simulink model "V2X_UDP_SCLX_Control_2019b"  (R2019b)
settings: Solver=FixedStepDiscrete  StartTime=0.0  StopTime=Inf  FixedStep=0.01  RelTol=1e-3
PostLoadFcn:
  | if any(exist('dsrtsu_mdlpostloadfcn', 'file') ~= 0), dsrtsu_mdlpostloadfcn('Execute', bdroot); end
InitFcn:
  | , if any(exist('rtifpga_mdlclblib', 'file') ~= 0), rtifpga_mdlclblib('Init', bdroot); end,
  | , if any(exist('dsmpb_private', 'file') ~= 0), dsmpb_private('dsmpb_mdlclblib', 'Init', bdroot); end,
values from neighbouring files (symbols this model uses):
  CtrlZone_Length = 250    [HDVPSG_DelayComp_NewRef_RealDrop_script_case1.m]
  High_TRFC = 1    [HDVPSG_DelayComp_NewRef_RealDrop_script_case1.m]
  PSG_AMAX = 3.2    [HDVPSG_DelayComp_NewRef_RealDrop_script_case1.m]
  PSG_AMIN = -6    [HDVPSG_DelayComp_NewRef_RealDrop_script_case1.m]
  PSG_first_v0 = 13    [HDVPSG_DelayComp_NewRef_RealDrop_script_case1.m]
  PSG_HighMu_D = 15    [HDVPSG_DelayComp_NewRef_RealDrop_script_case1.m]
  PSG_HighMu_I = 125    [HDVPSG_DelayComp_NewRef_RealDrop_script_case1.m]
  PSG_HighMu_P = 75    [HDVPSG_DelayComp_NewRef_RealDrop_script_case1.m]
  PSG_HighMu_TRFC = 0.8    [HDVPSG_DelayComp_NewRef_RealDrop_script_case1.m]
  PSG_LowMu_D = 12    [HDVPSG_DelayComp_NewRef_RealDrop_script_case1.m]
  PSG_LowMu_I = 64    [HDVPSG_DelayComp_NewRef_RealDrop_script_case1.m]
  PSG_LowMu_P = 48    [HDVPSG_DelayComp_NewRef_RealDrop_script_case1.m]
  PSG_LowMu_TRFC = 0.7    [HDVPSG_DelayComp_NewRef_RealDrop_script_case1.m]
  Q_Leader = 1    [HDVPSG_DelayComp_NewRef_RealDrop_script_case1.m]
  R_Leader = 20    [HDVPSG_DelayComp_NewRef_RealDrop_script_case1.m]
  T_ADE = 0.01    [HDVPSG_DelayComp_NewRef_RealDrop_script_case1.m]
  V_MAX = 40    [HDVPSG_DelayComp_NewRef_RealDrop_script_case1.m]
  V_MIN = 0    [HDVPSG_DelayComp_NewRef_RealDrop_script_case1.m]
undefined symbols (not defined in the file or in its folder): BETA_PSG_Leader, DiscIntNeverNeededParam, UT
libraries: simulink x4, dsmpblib x3
(part 2 of 3)

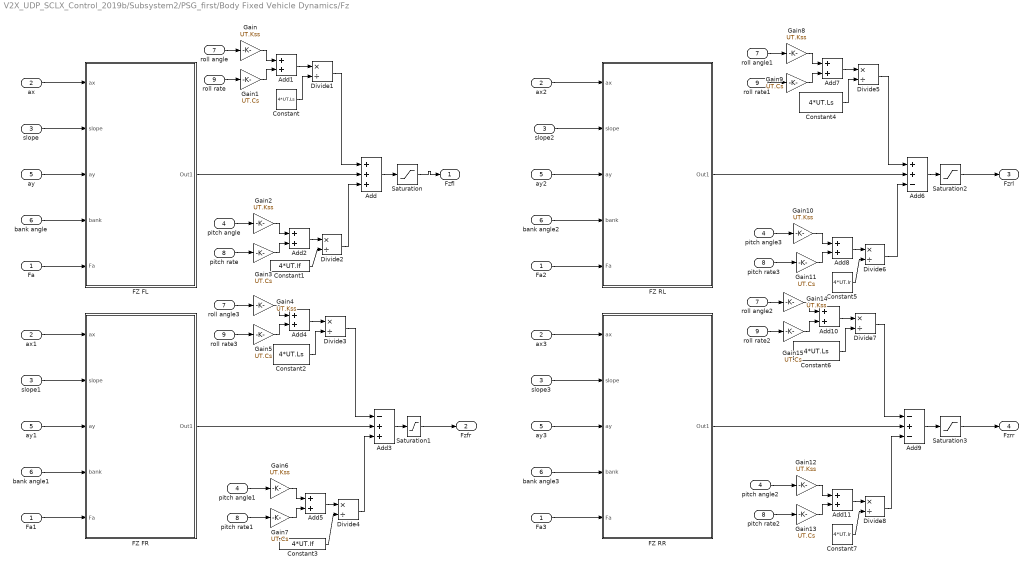
== system V2X_UDP_SCLX_Control_2019b/Subsystem2/PSG_first/Body Fixed Vehicle Dynamics/Fz ==
  Fa : Inport
  ax : Inport  Port=2
  slope : Inport  Port=3
  pitch angle : Inport  Port=4
  ay : Inport  Port=5
  bank angle : Inport  Port=6
  roll angle : Inport  Port=7
  pitch rate : Inport  Port=8
  roll rate : Inport  Port=9
  Add : Sum  Inputs=+++
  Add{1..2,4..5,7..8,10..11} (8 alike) : Sum
  Add3 : Sum  Inputs=-++
  Add6 : Sum  Inputs=++-
  Add9 : Sum  Inputs=-+-
  Constant{,2,4,6} (4 alike) : Constant  Value=4*UT.Ls
  Constant1 : Constant  Value=4*UT.lf
  Constant3 : Constant  Value=4*UT.lf
  Constant5 : Constant  Value=4*UT.lr
  Constant7 : Constant  Value=4*UT.lr
  Divide{1..8} (8 alike) : Product  Inputs=*/
  FZ FL : Subsystem
  FZ FR : Subsystem
  FZ RL : Subsystem
  FZ RR : Subsystem
  Fa1 : InportShadow
  Fa2 : InportShadow
  Fa3 : InportShadow
  Gain{,2,4,6,8,10,12,14} (8 alike) : Gain  Gain=UT.Kss
  Gain{1,3,5,7,9,11,13,15} (8 alike) : Gain  Gain=UT.Cs
  Saturation{,1..3} (4 alike) : Saturate  UpperLimit=10000  LowerLimit=100
  ax1 : InportShadow  Port=2
  ax2 : InportShadow  Port=2
  ax3 : InportShadow  Port=2
  ay1 : InportShadow  Port=5
  ay2 : InportShadow  Port=5
  ay3 : InportShadow  Port=5
  bank angle1 : InportShadow  Port=6
  bank angle2 : InportShadow  Port=6
  bank angle3 : InportShadow  Port=6
  pitch angle1 : InportShadow  Port=4
  pitch angle2 : InportShadow  Port=4
  pitch angle3 : InportShadow  Port=4
  pitch rate1 : InportShadow  Port=8
  pitch rate2 : InportShadow  Port=8
  pitch rate3 : InportShadow  Port=8
  roll angle1 : InportShadow  Port=7
  roll angle2 : InportShadow  Port=7
  roll angle3 : InportShadow  Port=7
  roll rate1 : InportShadow  Port=9
  roll rate2 : InportShadow  Port=9
  roll rate3 : InportShadow  Port=9
  slope1 : InportShadow  Port=3
  slope2 : InportShadow  Port=3
  slope3 : InportShadow  Port=3
  Fzfl : Outport  VectorParamsAs1DForOutWhenUnconnected=off
  Fzfr : Outport  Port=2  VectorParamsAs1DForOutWhenUnconnected=off
  Fzrl : Outport  Port=3  VectorParamsAs1DForOutWhenUnconnected=off
  Fzrr : Outport  Port=4  VectorParamsAs1DForOutWhenUnconnected=off
  wires:
  slope/1 -> FZ FL/2(slope)
  ax/1 -> FZ FL/1(ax)
  ay/1 -> FZ FL/3(ay)
  Fa/1 -> FZ FL/5(Fa)
  bank angle/1 -> FZ FL/4(bank)
  ay2/1 -> FZ RL/3(ay)
  slope2/1 -> FZ RL/2(slope)
  bank angle2/1 -> FZ RL/4(bank)
  ax2/1 -> FZ RL/1(ax)
  Fa2/1 -> FZ RL/5(Fa)
  slope3/1 -> FZ RR/2(slope)
  ay3/1 -> FZ RR/3(ay)
  Fa3/1 -> FZ RR/5(Fa)
  ax3/1 -> FZ RR/1(ax)
  bank angle3/1 -> FZ RR/4(bank)
  slope1/1 -> FZ FR/2(slope)
  ax1/1 -> FZ FR/1(ax)
  ay1/1 -> FZ FR/3(ay)
  bank angle1/1 -> FZ FR/4(bank)
  Fa1/1 -> FZ FR/5(Fa)
  roll angle/1 -> Gain/1
  roll rate/1 -> Gain1/1
  Gain1/1 -> Add1/2
  Gain/1 -> Add1/1
  Add1/1 -> Divide1/1
  Constant/1 -> Divide1/2
  FZ FL/1(Out1) -> Add/2
  Add/1 -> Saturation/1
  Gain3/1 -> Add2/2
  Gain2/1 -> Add2/1
  Add2/1 -> Divide2/1
  Constant1/1 -> Divide2/2
  pitch angle/1 -> Gain2/1
  pitch rate/1 -> Gain3/1
  roll angle3/1 -> Gain4/1
  roll rate3/1 -> Gain5/1
  Gain5/1 -> Add4/2
  Gain4/1 -> Add4/1
  Add4/1 -> Divide3/1
  Constant2/1 -> Divide3/2
  FZ FR/1(Out1) -> Add3/2
  Gain7/1 -> Add5/2
  Gain6/1 -> Add5/1
  Add5/1 -> Divide4/1
  Constant3/1 -> Divide4/2
  pitch angle1/1 -> Gain6/1
  pitch rate1/1 -> Gain7/1
  roll angle1/1 -> Gain8/1
  roll rate1/1 -> Gain9/1
  Gain9/1 -> Add7/2
  Gain8/1 -> Add7/1
  Add7/1 -> Divide5/1
  Constant4/1 -> Divide5/2
  FZ RL/1(Out1) -> Add6/2
  Gain11/1 -> Add8/2
  Gain10/1 -> Add8/1
  Add8/1 -> Divide6/1
  Constant5/1 -> Divide6/2
  pitch angle3/1 -> Gain10/1
  pitch rate3/1 -> Gain11/1
  roll angle2/1 -> Gain14/1
  roll rate2/1 -> Gain15/1
  Gain15/1 -> Add10/2
  Gain14/1 -> Add10/1
  Add10/1 -> Divide7/1
  Constant6/1 -> Divide7/2
  FZ RR/1(Out1) -> Add9/2
  Gain13/1 -> Add11/2
  Gain12/1 -> Add11/1
  Add11/1 -> Divide8/1
  Constant7/1 -> Divide8/2
  pitch angle2/1 -> Gain12/1
  pitch rate2/1 -> Gain13/1
  Add3/1 -> Saturation1/1
  Add6/1 -> Saturation2/1
  Add9/1 -> Saturation3/1
  Divide1/1 -> Add/1
  Divide3/1 -> Add3/1
  Divide5/1 -> Add6/1
  Divide7/1 -> Add9/1
  Saturation/1 -> Fzfl/1
  Saturation1/1 -> Fzfr/1
  Saturation2/1 -> Fzrl/1
  Saturation3/1 -> Fzrr/1
  Divide4/1 -> Add3/3
  Divide2/1 -> Add/3
  Divide8/1 -> Add9/3
  Divide6/1 -> Add6/3

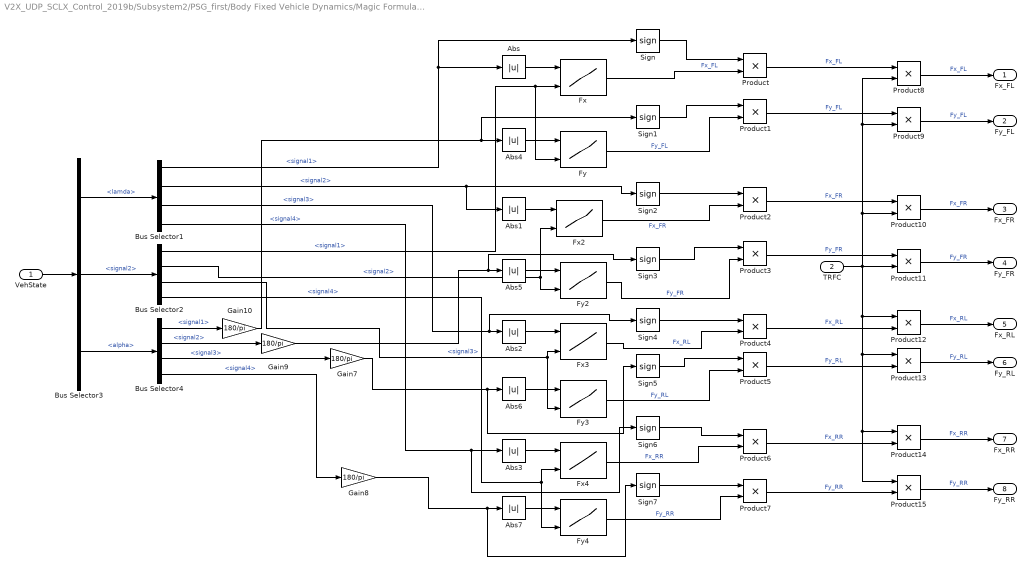
== system V2X_UDP_SCLX_Control_2019b/Subsystem2/PSG_first/Body Fixed Vehicle Dynamics/Magic Formula Tire Model1 ==
  VehState : Inport
  TRFC : Inport  Port=2
  Abs{,1..7} (8 alike) : Abs
  Bus Selector1 : BusSelector  OutputSignals=signal1,signal2,signal3,signal4
  Bus Selector2 : BusSelector  OutputSignals=signal1,signal2,signal3,signal4
  Bus Selector3 : BusSelector  OutputSignals=lamda,signal2,alpha
  Bus Selector4 : BusSelector  OutputSignals=signal1,signal2,signal3,signal4
  Fx{,2..4} (4 alike) : Lookup_n-D  BreakpointsForDimension1=[0,0.02,0.04,0.06,0.08,0.1,0.12,0.14,0.16,0.18,0.2,0.25,0.3,0.4,0.5,0.6,0.7,0.8,0.9,1]  BreakpointsForDimension2=[0,2105,3995,6120,7900,10100]  Table=reshape([0,0,0,0,0,0,0,0,0,0,0,0,0,0,0,0,0,0,0,0,0,926.741,1701.43,2240.07,2548.95,2689.78,2729.82,2717.36,2680.7,2634.75,2586.89,2476.95,2388.22,2262.94,2181.64,2125.47,2084.58,2053.55,2029.26,2029.26,0,1853.48,3402.86,4480.13,5097.92,5379.54,5459.63,5434.73,5361.4,5269.5,5173.78,4953.9,4776.46,4525.87,4363.28,4250.95,4169.16,4107.12,4058.51,4058.51,0,2780.22,5104.29,6720.21,7646.88,8069.32,8189.45,8152.09,8042.1,7904.24,7760.68,7430.85,7164.69,6788.82,6544.93,6376.42,6253.75,6160.67,6087.76,6087.76,0,3706.97,6805.72,8960.27,10195.8,10759.1,10919.3,10869.4,10722.8,10539,10347.6,9907.79,9552.92,9051.76,8726.56,8501.91,8338.33,8214.24,8117.01,8117.01,0,4633.7,8507.15,11200.3,12744.8,13448.8,13649.1,13586.8,13403.5,13173.7,12934.4,12384.7,11941.1,11314.7,10908.2,10627.4,10422.9,10267.8,10146.3,10146.3],20,6)  RndMeth=Simplest  InputSameDT=on
  Fy{,2..4} (4 alike) : Lookup_n-D  BreakpointsForDimension1=[0,0.5,1,1.5,2,2.5,3,3.5,4,4.5,5,5.5,6,6.5,7,7.5,8,8.5,9,9.5,10,12,14,16,18,20]  BreakpointsForDimension2=[0,1725,3500,6100,6950,9005]  Table=reshape([0,0,0,0,0,0,0,0,0,0,0,0,0,0,0,0,0,0,0,0,0,0,0,0,0,0,0,444.357,843.546,1162.09,1403.45,1580.72,1707.08,1795.66,1859.6,1893.83,1904.16,1896.19,1875.03,1845.3,1810.95,1775.12,1740.18,1707.8,1678.67,1653.27,1631.62,1574.53,1546.58,1531.91,1523.64,1523.64,0,894.186,1694.5,2327.41,2800.6,3142.1,3379.93,3542.12,3656.67,3713.24,3724.46,3701.92,3656.45,3597,3531.15,3464.91,3402.12,3345.23,3295.32,3252.61,3216.48,3123.37,3078,3054.18,3040.4,3040.4,0,1293.54,2452.99,3373.13,4064.18,4565.24,4915.41,5153.78,5319.43,5402.64,5422.23,5395.45,5337.38,5261.2,5177.14,5092.89,5013.56,4942.1,4879.5,4825.96,4780.78,4662.96,4604.6,4573.3,4554.99,4554.99,0,1601.93,3047.78,4214.48,5111.02,5779.43,6261.69,6599.82,6835.85,6968.31,7019.99,7011.91,6962.7,6887.9,6800.2,6709.15,6621.16,6540.06,6467.91,6405.21,6351.47,6207.67,6133.95,6093.89,6070.17,6070.17,0,1784.39,3417.9,4780.29,5873.77,6731.16,7385.32,7869.06,8215.23,8439.3,8564.79,8613.61,8605.54,8557.9,8485.17,8398.94,8308.19,8219.02,8135.36,8059.17,7991.56,7798.93,7693.72,7634.76,7599.62,7599.62],26,6)  RndMeth=Simplest  InputSameDT=on
  Gain{7..10} (4 alike) : Gain  Gain=180/pi  SaturateOnIntegerOverflow=on  SampleTime=UT.Ts_Veh  OutDataTypeStr=Inherit: Same as input  ParamDataTypeStr=Inherit: Same as input
  Product{,1..15} (16 alike) : Product
  Sign{,1..7} (8 alike) : Signum
  Fx_FL : Outport  VectorParamsAs1DForOutWhenUnconnected=off
  Fy_FL : Outport  Port=2  VectorParamsAs1DForOutWhenUnconnected=off
  Fx_FR : Outport  Port=3  VectorParamsAs1DForOutWhenUnconnected=off
  Fy_FR : Outport  Port=4  VectorParamsAs1DForOutWhenUnconnected=off
  Fx_RL : Outport  Port=5  VectorParamsAs1DForOutWhenUnconnected=off
  Fy_RL : Outport  Port=6  VectorParamsAs1DForOutWhenUnconnected=off
  Fx_RR : Outport  Port=7  VectorParamsAs1DForOutWhenUnconnected=off
  Fy_RR : Outport  Port=8  VectorParamsAs1DForOutWhenUnconnected=off
  wires:
  TRFC/1 -> Product11/2, Product10/2, Product9/2, Product8/2, Product12/1, Product13/1, Product14/1, Product15/1
  Product1/1 -> Product9/1  "Fy_FL"
  Product7/1 -> Product15/2  "Fy_RR"
  Product5/1 -> Product13/2  "Fy_RL"
  Product3/1 -> Product11/1  "Fy_FR"
  Bus Selector3/3 -> Bus Selector4/1  "<alpha>"
  Bus Selector3/2 -> Bus Selector2/1  "<signal2>"
  Bus Selector3/1 -> Bus Selector1/1  "<lamda>"
  Bus Selector4/4 -> Gain8/1  "<signal4>"
  Bus Selector4/3 -> Gain7/1  "<signal3>"
  Bus Selector4/2 -> Gain9/1  "<signal2>"
  Bus Selector4/1 -> Gain10/1  "<signal1>"
  Bus Selector1/4 -> Sign6/1, Abs3/1  "<signal4>"
  VehState/1 -> Bus Selector3/1
  Bus Selector1/1 -> Sign/1, Abs/1  "<signal1>"
  Bus Selector1/2 -> Sign2/1, Abs1/1  "<signal2>"
  Bus Selector1/3 -> Sign4/1, Abs2/1  "<signal3>"
  Abs/1 -> Fx/1
  Bus Selector2/1 -> Fy/2, Fx/2  "<signal1>"
  Abs1/1 -> Fx2/1
  Abs2/1 -> Fx3/1
  Bus Selector2/2 -> Fy2/2, Fx2/2  "<signal2>"
  Bus Selector2/3 -> Fy3/2, Fx3/2  "<signal3>"
  Abs3/1 -> Fx4/1
  Bus Selector2/4 -> Fy4/2, Fx4/2  "<signal4>"
  Abs4/1 -> Fy/1
  Abs5/1 -> Fy2/1
  Abs6/1 -> Fy3/1
  Abs7/1 -> Fy4/1
  Gain10/1 -> Sign1/1, Abs4/1
  Gain9/1 -> Sign3/1, Abs5/1
  Gain7/1 -> Sign5/1, Abs6/1
  Gain8/1 -> Sign7/1, Abs7/1
  Sign/1 -> Product/1
  Fx/1 -> Product/2  "Fx_FL"
  Product/1 -> Product8/1  "Fx_FL"
  Sign1/1 -> Product1/1
  Fy/1 -> Product1/2  "Fy_FL"
  Sign2/1 -> Product2/1
  Fx2/1 -> Product2/2  "Fx_FR"
  Product2/1 -> Product10/1  "Fx_FR"
  Sign3/1 -> Product3/1
  Fy2/1 -> Product3/2  "Fy_FR"
  Sign4/1 -> Product4/1
  Fx3/1 -> Product4/2  "Fx_RL"
  Product4/1 -> Product12/2  "Fx_RL"
  Sign5/1 -> Product5/1
  Fy3/1 -> Product5/2  "Fy_RL"
  Sign6/1 -> Product6/1
  Fx4/1 -> Product6/2  "Fx_RR"
  Product6/1 -> Product14/2  "Fx_RR"
  Sign7/1 -> Product7/1
  Fy4/1 -> Product7/2  "Fy_RR"
  Product8/1 -> Fx_FL/1  "Fx_FL"
  Product9/1 -> Fy_FL/1  "Fy_FL"
  Product10/1 -> Fx_FR/1  "Fx_FR"
  Product11/1 -> Fy_FR/1  "Fy_FR"
  Product12/1 -> Fx_RL/1  "Fx_RL"
  Product13/1 -> Fy_RL/1  "Fy_RL"
  Product14/1 -> Fx_RR/1  "Fx_RR"
  Product15/1 -> Fy_RR/1  "Fy_RR"

== system V2X_UDP_SCLX_Control_2019b/Subsystem2/PSG_first/Body Fixed Vehicle Dynamics/Tire Longitudinal Center Speed  ==
  note: Vcg
  Vx : Inport
  Vy : Inport  Port=2
  YawRate : Inport  Port=3
  VehSideSlip Beta : Inport  Port=4
  Add{,1,4,6,8} (5 alike) : Sum  SampleTime=UT.Ts_Veh
  Add2 : Sum  Inputs=+-  SampleTime=UT.Ts_Veh
  Add3 : Sum  Inputs=-+  SampleTime=UT.Ts_Veh
  Add5 : Sum  Inputs=-+  SampleTime=UT.Ts_Veh
  Add7 : Sum  Inputs=+-  SampleTime=UT.Ts_Veh
  Gain : Gain
  "Ls " : Constant  Value=UT.Ls
  Math Function : Math  Operator=square  SignedPower=on  SampleTime=UT.Ts_Veh  SaturateOnIntegerOverflow=on
  Math Function1 : Math  Operator=square  SignedPower=on  SampleTime=UT.Ts_Veh  SaturateOnIntegerOverflow=on
  Product{,1..5} (6 alike) : Product  SampleTime=UT.Ts_Veh
  Sqrt : Sqrt  SampleTime=UT.Ts_Veh  SaturateOnIntegerOverflow=on
  lf : Constant  Value=UT.lf
  lr : Constant  Value=UT.lr
  Vwfl : Outport  VectorParamsAs1DForOutWhenUnconnected=off
  Vwfr : Outport  Port=2  VectorParamsAs1DForOutWhenUnconnected=off
  Vwrl : Outport  Port=3  VectorParamsAs1DForOutWhenUnconnected=off
  Vwrr : Outport  Port=4  VectorParamsAs1DForOutWhenUnconnected=off
  wires:
  Vy/1 -> Math Function1/1
  Vx/1 -> Math Function/1
  Math Function/1 -> Add/1
  Math Function1/1 -> Add/2
  Add/1 -> Sqrt/1
  YawRate/1 -> Product5/1, Product4/1, Product2/1, Product1/1
  lf/1 -> Product/2
  VehSideSlip Beta/1 -> Gain/1
  Product/1 -> Add4/1, Add3/1
  "Ls "/1 -> Add5/2, Add6/1, Add4/2, Add3/2
  Add3/1 -> Product1/2
  Sqrt/1 -> Add8/1, Add7/1, Add1/1, Add2/1
  Product1/1 -> Add2/2
  Add2/1 -> Vwfl/1
  Add4/1 -> Product2/2
  Product2/1 -> Add1/2
  Add1/1 -> Vwfr/1
  lr/1 -> Product3/2
  Product3/1 -> Add5/1, Add6/2
  Add6/1 -> Product4/2
  Product4/1 -> Add7/2
  Add7/1 -> Vwrl/1
  Add5/1 -> Product5/2
  Product5/1 -> Add8/2
  Add8/1 -> Vwrr/1
  Gain/1 -> Product/1, Product3/1

== system V2X_UDP_SCLX_Control_2019b/Subsystem2/PSG_first/Body Fixed Vehicle Dynamics/Tire Sideslip Angle ==
  Vy : Inport
  Yaw Rate : Inport  Port=2
  Vx : Inport  Port=3
  deltaFL : Inport  Port=4
  deltaFR1 : Inport  Port=5
  Beta : Inport  Port=6
  Add : Sum  SampleTime=UT.Ts_Veh
  Add1 : Sum  Inputs=--+  SampleTime=UT.Ts_Veh
  Add2 : Sum  Inputs=-+  SampleTime=UT.Ts_Veh
  Add4 : Sum  Inputs=--+  SampleTime=UT.Ts_Veh
  Constant : Constant  Value=UT.lf
  Constant1 : Constant  Value=UT.lr
  Constant2 : Constant  Value=0.001
  Constant{3..6} (4 alike) : Constant  Value=0
  Divide : Product  Inputs=*/  SampleTime=UT.Ts_Veh
  Divide1 : Product  Inputs=/*  SampleTime=UT.Ts_Veh
  Gain{8..11} (4 alike) : Gain
  Math Function : Math  Operator=square  SignedPower=on  SampleTime=UT.Ts_Veh  SaturateOnIntegerOverflow=on
  Math Function1 : Math  Operator=square  SignedPower=on  SampleTime=UT.Ts_Veh  SaturateOnIntegerOverflow=on
  Product : Product  SampleTime=UT.Ts_Veh
  Product1 : Product  SampleTime=UT.Ts_Veh
  Saturation : Saturate  UpperLimit=1  LowerLimit=-1
  Saturation{1,3..5} (4 alike) : Saturate  UpperLimit=15*3.14/180  LowerLimit=-15*3.14/180
  Saturation2 : Saturate  UpperLimit=1  LowerLimit=-1
  Sqrt : Sqrt  SampleTime=UT.Ts_Veh  SaturateOnIntegerOverflow=on
  Switch : Switch  Criteria=u2 > Threshold
  Switch{1..4} (4 alike) : Switch  Threshold=2
  Vx{1..4} (4 alike) : InportShadow  Port=3
  Yaw Rate1 : InportShadow  Port=2
  alpha_fl: rad : Outport  VectorParamsAs1DForOutWhenUnconnected=off
  alpha_fr: rad : Outport  Port=2  VectorParamsAs1DForOutWhenUnconnected=off
  alpha_rl: rad : Outport  Port=3  VectorParamsAs1DForOutWhenUnconnected=off
  alpha_rr: rad : Outport  Port=4  VectorParamsAs1DForOutWhenUnconnected=off
  wires:
  Constant/1 -> Product/2
  Yaw Rate/1 -> Product/1
  Product/1 -> Divide/1
  Constant1/1 -> Product1/2
  Add1/1 -> Saturation/1
  Vx/1 -> Math Function1/1
  Add4/1 -> Saturation2/1
  Constant4/1 -> Switch3/3
  Vx1/1 -> Switch3/2
  Switch3/1 -> Saturation1/1
  Constant3/1 -> Switch1/3
  Vx2/1 -> Switch1/2
  Switch1/1 -> Saturation5/1
  Constant5/1 -> Switch2/3
  Vx3/1 -> Switch2/2
  Switch2/1 -> Saturation3/1
  Constant6/1 -> Switch4/3
  Vx4/1 -> Switch4/2
  Switch4/1 -> Saturation4/1
  Saturation1/1 -> Gain9/1
  Saturation5/1 -> Gain8/1
  Saturation3/1 -> Gain10/1
  Saturation4/1 -> Gain11/1
  Gain9/1 -> alpha_fl: rad/1
  Gain8/1 -> alpha_fr: rad/1
  Gain10/1 -> alpha_rl: rad/1
  Gain11/1 -> alpha_rr: rad/1
  deltaFL/1 -> Add1/3
  Math Function/1 -> Add/1
  Math Function1/1 -> Add/2
  Add/1 -> Sqrt/1
  Vy/1 -> Math Function/1
  Saturation/1 -> Switch3/1
  Divide/1 -> Add1/2, Add4/2
  deltaFR1/1 -> Add4/3
  Beta/1 -> Add2/1, Add4/1, Add1/1
  Saturation2/1 -> Switch1/1
  Divide1/1 -> Add2/2
  Add2/1 -> Switch4/1, Switch2/1
  Sqrt/1 -> Switch/2, Switch/1
  Constant2/1 -> Switch/3
  Switch/1 -> Divide/2, Divide1/1
  Product1/1 -> Divide1/2
  Yaw Rate1/1 -> Product1/1

== system V2X_UDP_SCLX_Control_2019b/Subsystem2/PSG_first/Body Fixed Vehicle Dynamics/lamda slip ratio ==
  note: used to be divided by the max of abs of wheel vel or vwcosdelta
  omegafl : Inport
  omegafr : Inport  Port=2
  omegarl : Inport  Port=3
  omegarr : Inport  Port=4
  Vwfl : Inport  Port=5
  Vwfr : Inport  Port=6
  Vwrl : Inport  Port=7
  Vwrr : Inport  Port=8
  deltaFL : Inport  Port=9
  deltaFR : Inport  Port=10
  Abs{,1..7} (8 alike) : Abs
  Constant : Constant  Value=UT.Rw
  Divide : Product  Inputs=*/  SampleTime=UT.Ts_Veh
  Divide1 : Product  Inputs=*/
  Divide2 : Product  Inputs=*/
  Divide3 : Product  Inputs=*/  SampleTime=UT.Ts_Veh
  Gain{,1..3} (4 alike) : Gain  Gain=0.1
  MinMax{,1..3} (4 alike) : MinMax  Function=max  Inputs=2
  Product{,1..5} (6 alike) : Product  SampleTime=UT.Ts_Veh
  Subtract : Sum  Inputs=+-  SampleTime=UT.Ts_Veh
  Subtract1 : Sum  Inputs=+-
  Subtract2 : Sum  Inputs=+-  SampleTime=UT.Ts_Veh
  Subtract3 : Sum  Inputs=+-  SampleTime=UT.Ts_Veh
  Trigonometric Function : Trigonometry  Operator=cos  SampleTime=UT.Ts_Veh
  Trigonometric Function1 : Trigonometry  Operator=cos
  lamdafl : Outport  VectorParamsAs1DForOutWhenUnconnected=off
  lamdafr : Outport  Port=2  VectorParamsAs1DForOutWhenUnconnected=off
  lamdarl : Outport  Port=3  VectorParamsAs1DForOutWhenUnconnected=off
  lamdarr : Outport  Port=4  VectorParamsAs1DForOutWhenUnconnected=off
  wires:
  omegafl/1 -> Product/1
  omegafr/1 -> Product1/1
  omegarl/1 -> Product2/1
  omegarr/1 -> Product3/1
  Constant/1 -> Product1/2, Product/2, Product3/2, Product2/2
  Product/1 -> Abs/1, Subtract/1
  Product1/1 -> Abs2/1, Subtract1/1
  Product2/1 -> Abs4/1, Subtract2/1
  Product3/1 -> Abs6/1, Subtract3/1
  Trigonometric Function/1 -> Product4/2
  Divide/1 -> Gain/1  "lamda_FL"
  Trigonometric Function1/1 -> Product5/2
  Vwfr/1 -> Product5/1
  Product5/1 -> Subtract1/2, Abs3/1
  Vwfl/1 -> Product4/1
  Vwrl/1 -> Abs5/1, Subtract2/2
  Subtract/1 -> Divide/1
  Subtract1/1 -> Divide1/1
  Subtract2/1 -> Divide2/1
  Subtract3/1 -> Divide3/1
  Abs/1 -> MinMax/1
  Abs1/1 -> MinMax/2
  MinMax/1 -> Divide/2
  Abs2/1 -> MinMax1/1
  Abs3/1 -> MinMax1/2
  MinMax1/1 -> Divide1/2
  Abs4/1 -> MinMax2/1
  Abs5/1 -> MinMax2/2
  MinMax2/1 -> Divide2/2
  Abs6/1 -> MinMax3/1
  Abs7/1 -> MinMax3/2
  MinMax3/1 -> Divide3/2
  Divide2/1 -> Gain2/1  "lamda_RL"
  Divide3/1 -> Gain3/1  "lamda_RR"
  Divide1/1 -> Gain1/1  "lamda_FR"
  Gain/1 -> lamdafl/1
  Gain2/1 -> lamdarl/1
  Vwrr/1 -> Abs7/1, Subtract3/2
  deltaFL/1 -> Trigonometric Function/1
  deltaFR/1 -> Trigonometric Function1/1
  Product4/1 -> Subtract/2, Abs1/1
  Gain1/1 -> lamdafr/1
  Gain3/1 -> lamdarr/1

== system V2X_UDP_SCLX_Control_2019b/Subsystem2/PSG_first/Body Fixed Vehicle Dynamics/8dof_vehicle/4tyre_torque ==
  note: -20/Rw
  Tdf : Inport
  Tbfl : Inport  Port=2
  Tbfr : Inport  Port=3
  Tbrl : Inport  Port=4
  Tbrr : Inport  Port=5
  Fxfl : Inport  Port=6
  Fxfr : Inport  Port=7
  Fxrl : Inport  Port=8
  Fxrr : Inport  Port=9
  V_ini : Inport  Port=10
  Add2 : Sum  Inputs=--+
  Add3 : Sum  Inputs=+--
  Add4 : Sum  Inputs=--
  Add5 : Sum  Inputs=--
  Constant{,1..4} (5 alike) : Constant  Value=UT.Rw
  Discrete-Time Integrator{,1..3} (4 alike) : DiscreteIntegrator  InitialConditionSource=external  InitialCondition=UT.Veh_PSG_o(7)  SampleTime=UT.Ts_Veh  ICPrevOutput=DiscIntNeverNeededParam  ICPrevScaledInput=DiscIntNeverNeededParam
  Divide{,1..3} (4 alike) : Product  Inputs=*/
  Gain{1..3,5} (4 alike) : Gain  Gain=1/UT.Jw
  Product{,1..3} (4 alike) : Product
  Saturation{,1..3} (4 alike) : Saturate  UpperLimit=100/UT.Rw  LowerLimit=-20/UT.Rw
  omega_fl : Outport  VectorParamsAs1DForOutWhenUnconnected=off
  omega_fr : Outport  Port=2  VectorParamsAs1DForOutWhenUnconnected=off
  omega_rl : Outport  Port=3  VectorParamsAs1DForOutWhenUnconnected=off
  omega_rr : Outport  Port=4  VectorParamsAs1DForOutWhenUnconnected=off
  wires:
  V_ini/1 -> Divide/1, Divide1/1, Divide2/1, Divide3/1
  Divide3/1 -> Discrete-Time Integrator3/2
  Constant4/1 -> Divide3/2
  Constant3/1 -> Divide2/2
  Divide2/1 -> Discrete-Time Integrator2/2
  Divide1/1 -> Discrete-Time Integrator1/2
  Constant2/1 -> Divide1/2
  Constant1/1 -> Divide/2
  Divide/1 -> Discrete-Time Integrator/2
  Tbrr/1 -> Add5/1
  Tbfr/1 -> Add3/2
  Product1/1 -> Add3/3
  Saturation3/1 -> omega_rr/1
  Saturation2/1 -> omega_rl/1
  Saturation1/1 -> omega_fr/1
  Saturation/1 -> omega_fl/1
  Fxrr/1 -> Product3/2
  Fxrl/1 -> Product2/2
  Fxfr/1 -> Product1/2
  Fxfl/1 -> Product/1
  Gain5/1 -> Discrete-Time Integrator/1
  Add5/1 -> Gain3/1
  Add4/1 -> Gain2/1
  Add2/1 -> Gain5/1
  Add3/1 -> Gain1/1
  Tbrl/1 -> Add4/1
  Discrete-Time Integrator3/1 -> Saturation3/1
  Discrete-Time Integrator2/1 -> Saturation2/1
  Gain2/1 -> Discrete-Time Integrator2/1
  Discrete-Time Integrator1/1 -> Saturation1/1
  Gain1/1 -> Discrete-Time Integrator1/1
  Discrete-Time Integrator/1 -> Saturation/1
  Tbfl/1 -> Add2/2
  Product2/1 -> Add4/2
  Product3/1 -> Add5/2
  Constant/1 -> Product1/1, Product2/1, Product3/1, Product/2
  Tdf/1 -> Add2/3, Add3/1
  Product/1 -> Add2/1
  Gain3/1 -> Discrete-Time Integrator3/1

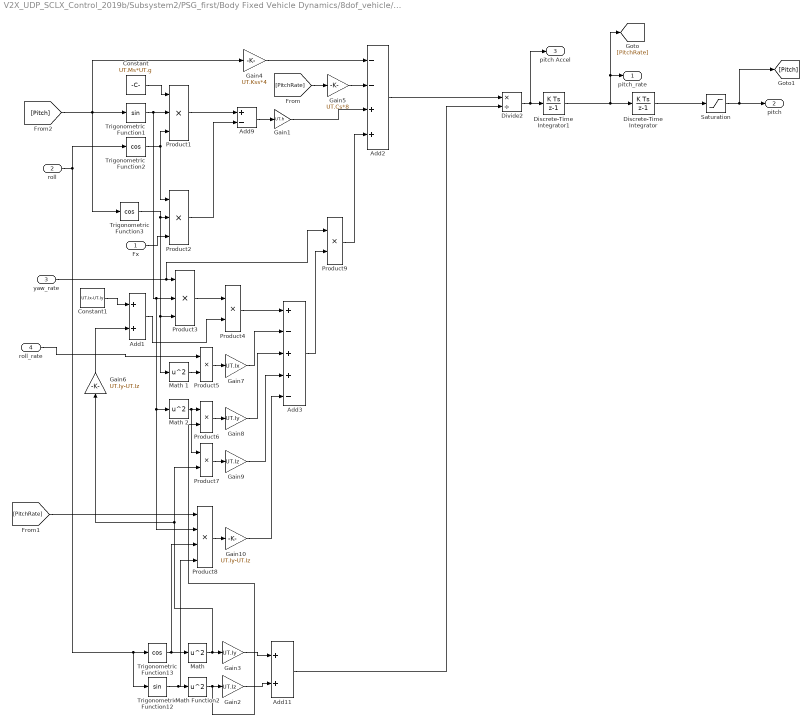
== system V2X_UDP_SCLX_Control_2019b/Subsystem2/PSG_first/Body Fixed Vehicle Dynamics/8dof_vehicle/Pitch  ==
  Fx : Inport
  roll : Inport  Port=2
  yaw_rate : Inport  Port=3
  roll_rate : Inport  Port=4
  Add1 : Sum
  Add11 : Sum
  Add2 : Sum  Inputs=--++
  Add3 : Sum  Inputs=+-++-
  Add9 : Sum  Inputs=+-
  Constant : Constant  Value=UT.Ms*UT.g
  Constant1 : Constant  Value=UT.Ix-UT.Iy
  Discrete-Time Integrator : DiscreteIntegrator  SampleTime=UT.Ts_Veh  ICPrevOutput=DiscIntNeverNeededParam  ICPrevScaledInput=DiscIntNeverNeededParam
  Discrete-Time Integrator1 : DiscreteIntegrator  SampleTime=UT.Ts_Veh  ICPrevOutput=DiscIntNeverNeededParam  ICPrevScaledInput=DiscIntNeverNeededParam
  Divide2 : Product  Inputs=*/
  Gain1 : Gain  Gain=UT.h
  Gain10 : Gain  Gain=UT.Iy-UT.Iz
  Gain2 : Gain  Gain=UT.Iz
  Gain3 : Gain  Gain=UT.Iy
  Gain4 : Gain  Gain=UT.Kss*4
  Gain5 : Gain  Gain=UT.Cs*8
  Gain6 : Gain  Gain=UT.Iy-UT.Iz
  Gain7 : Gain  Gain=UT.Ix
  Gain8 : Gain  Gain=UT.Iy
  Gain9 : Gain  Gain=UT.Iz
  "Math " : Math  Operator=square  SignedPower=on  SaturateOnIntegerOverflow=on
  Math 1 : Math  Operator=square  SignedPower=on  SaturateOnIntegerOverflow=on
  Math 2 : Math  Operator=square  SignedPower=on  SaturateOnIntegerOverflow=on
  Math Function2 : Math  Operator=square  SignedPower=on  SaturateOnIntegerOverflow=on
  Product1 : Product  Inputs=3
  Product2 : Product  Inputs=3
  Product3 : Product  Inputs=3
  Product{4..7,9} (5 alike) : Product
  Product8 : Product  Inputs=4
  Saturation : Saturate  UpperLimit=0.18  LowerLimit=-0.18
  Trigonometric Function1 : Trigonometry
  Trigonometric Function12 : Trigonometry
  Trigonometric Function13 : Trigonometry  Operator=cos
  Trigonometric Function2 : Trigonometry  Operator=cos
  Trigonometric Function3 : Trigonometry  Operator=cos
  pitch_rate : Outport  VectorParamsAs1DForOutWhenUnconnected=off
  pitch : Outport  Port=2  VectorParamsAs1DForOutWhenUnconnected=off
  pitch Accel : Outport  Port=3  VectorParamsAs1DForOutWhenUnconnected=off
  wires:
  Saturation/1 -> [Pitch], pitch/1
  Discrete-Time Integrator1/1 -> [PitchRate], pitch_rate/1, Discrete-Time Integrator/1
  roll/1 -> Trigonometric Function12/1, Trigonometric Function13/1, Trigonometric Function2/1
  Add9/1 -> Gain1/1
  Trigonometric Function13/1 -> Product8/3, "Math "/1
  "Math "/1 -> Product7/2, Gain6/1, Gain3/1
  Gain3/1 -> Add11/1
  Trigonometric Function12/1 -> Product8/4, Math Function2/1
  Gain2/1 -> Add11/2
  Add11/1 -> Divide2/2
  [Pitch] -> Gain4/1, Trigonometric Function3/1, Trigonometric Function1/1
  Constant/1 -> Product1/1
  Trigonometric Function2/1 -> Product1/3, Product2/1
  Product1/1 -> Add9/1
  Fx/1 -> Product2/3
  Trigonometric Function3/1 -> Math 1/1, Product3/3, Product2/2
  Product2/1 -> Add9/2
  Gain1/1 -> Add2/3
  Gain4/1 -> Add2/1
  Gain5/1 -> Add2/2
  Divide2/1 -> pitch Accel/1, Discrete-Time Integrator1/1
  [PitchRate] -> Gain5/1
  yaw_rate/1 -> Product9/1, Product3/1
  Product3/1 -> Product4/1
  Constant1/1 -> Add1/1
  Gain6/1 -> Add1/2
  Add1/1 -> Product4/2
  Product4/1 -> Add3/1
  roll_rate/1 -> Product5/1
  Math 1/1 -> Product5/2
  Product5/1 -> Gain7/1
  Gain7/1 -> Add3/2
  Product6/1 -> Gain8/1
  Math 2/1 -> Product7/1, Product6/1
  Trigonometric Function1/1 -> Product1/2, Product8/2, Math 2/1, Product3/2
  Gain8/1 -> Add3/3
  Math Function2/1 -> Product6/2, Gain2/1
  Product7/1 -> Gain9/1
  Gain9/1 -> Add3/4
  Product8/1 -> Gain10/1
  [PitchRate] -> Product8/1
  Gain10/1 -> Add3/5
  Add3/1 -> Product9/2
  Product9/1 -> Add2/4
  Add2/1 -> Divide2/1
  Discrete-Time Integrator/1 -> Saturation/1

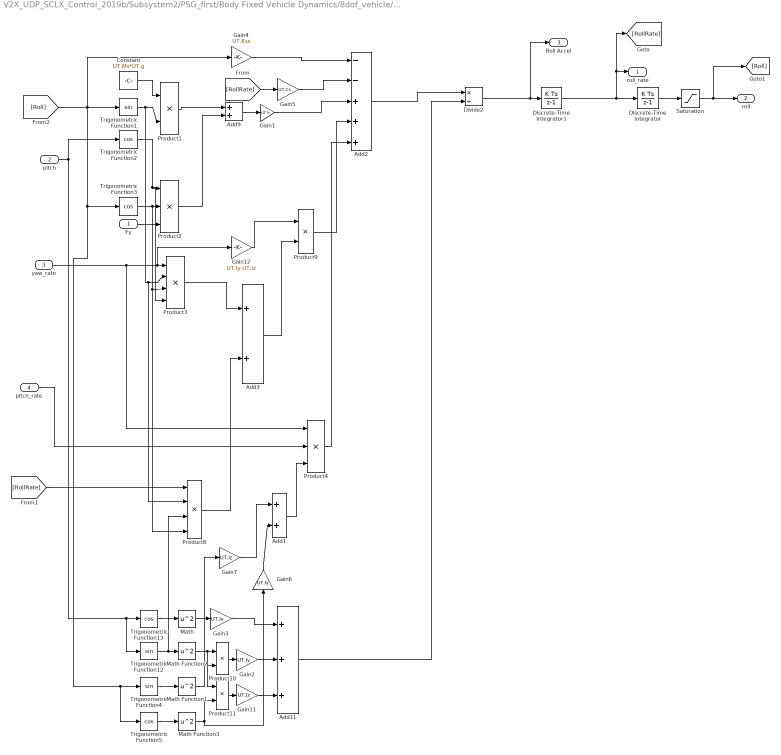
== system V2X_UDP_SCLX_Control_2019b/Subsystem2/PSG_first/Body Fixed Vehicle Dynamics/8dof_vehicle/Roll ==
  Fy : Inport
  pitch : Inport  Port=2
  yaw_rate : Inport  Port=3
  pitch_rate : Inport  Port=4
  Add1 : Sum
  Add11 : Sum  Inputs=+++
  Add2 : Sum  Inputs=--+++
  Add3 : Sum
  Add9 : Sum
  Constant : Constant  Value=UT.Ms*UT.g
  Discrete-Time Integrator : DiscreteIntegrator  SampleTime=UT.Ts_Veh  ICPrevOutput=DiscIntNeverNeededParam  ICPrevScaledInput=DiscIntNeverNeededParam
  Discrete-Time Integrator1 : DiscreteIntegrator  SampleTime=UT.Ts_Veh  ICPrevOutput=DiscIntNeverNeededParam  ICPrevScaledInput=DiscIntNeverNeededParam
  Divide2 : Product  Inputs=*/
  Gain1 : Gain  Gain=UT.h
  Gain11 : Gain  Gain=UT.Iz
  Gain12 : Gain  Gain=UT.Iy-UT.Iz
  Gain2 : Gain  Gain=UT.Iy
  Gain3 : Gain  Gain=UT.Ix
  Gain4 : Gain  Gain=UT.Kss
  Gain5 : Gain  Gain=UT.Cs
  Gain6 : Gain  Gain=UT.Iy
  Gain7 : Gain  Gain=UT.Iz
  "Math " : Math  Operator=square  SignedPower=on  SaturateOnIntegerOverflow=on
  Math Function1 : Math  Operator=square  SignedPower=on  SaturateOnIntegerOverflow=on
  Math Function2 : Math  Operator=square  SignedPower=on  SaturateOnIntegerOverflow=on
  Math Function3 : Math  Operator=square  SignedPower=on  SaturateOnIntegerOverflow=on
  Product{1,9..11} (4 alike) : Product
  Product2 : Product  Inputs=3
  Product3 : Product  Inputs=4
  Product4 : Product  Inputs=3
  Product8 : Product  Inputs=4
  Saturation : Saturate  UpperLimit=45  LowerLimit=-45
  Trigonometric Function1 : Trigonometry
  Trigonometric Function12 : Trigonometry
  Trigonometric Function{2..3,5,13} (4 alike) : Trigonometry  Operator=cos
  Trigonometric Function4 : Trigonometry
  roll_rate : Outport  VectorParamsAs1DForOutWhenUnconnected=off
  roll : Outport  Port=2  VectorParamsAs1DForOutWhenUnconnected=off
  Roll Accel : Outport  Port=3  VectorParamsAs1DForOutWhenUnconnected=off
  wires:
  Add2/1 -> Divide2/1
  Product9/1 -> Add2/4
  Add3/1 -> Product9/2
  [RollRate] -> Product8/1
  Product8/1 -> Add3/2
  Math Function2/1 -> Product11/1, Product10/1
  Trigonometric Function1/1 -> Product3/2, Product8/2, Product1/2
  Product3/1 -> Add3/1
  yaw_rate/1 -> Product4/1, Product3/1, Gain12/1
  [RollRate] -> Gain5/1
  Gain5/1 -> Add2/2
  Gain4/1 -> Add2/1
  Gain1/1 -> Add2/3
  Product2/1 -> Add9/2
  Trigonometric Function3/1 -> Product2/2, Product8/4, Product3/3
  Fy/1 -> Product2/3
  Product1/1 -> Add9/1
  Trigonometric Function2/1 -> Product3/4, Product2/1
  Constant/1 -> Product1/1
  [Roll] -> Trigonometric Function1/1, Trigonometric Function5/1, Trigonometric Function4/1, Trigonometric Function3/1, Gain4/1
  Add11/1 -> Divide2/2
  Trigonometric Function12/1 -> Product8/3, Math Function2/1
  Gain3/1 -> Add11/1
  "Math "/1 -> Gain3/1
  Trigonometric Function13/1 -> "Math "/1
  Add9/1 -> Gain1/1
  pitch/1 -> Trigonometric Function2/1, Trigonometric Function13/1, Trigonometric Function12/1
  Discrete-Time Integrator/1 -> Saturation/1
  Saturation/1 -> roll/1, [Roll]
  Product10/1 -> Gain2/1
  Trigonometric Function4/1 -> Math Function1/1
  Math Function1/1 -> Gain7/1, Product10/2
  Gain2/1 -> Add11/2
  Gain11/1 -> Add11/3
  Product11/1 -> Gain11/1
  Trigonometric Function5/1 -> Math Function3/1
  Math Function3/1 -> Product11/2, Gain6/1
  Gain12/1 -> Product9/1
  pitch_rate/1 -> Product4/2
  Gain6/1 -> Add1/2
  Gain7/1 -> Add1/1
  Add1/1 -> Product4/3
  Product4/1 -> Add2/5
  Divide2/1 -> Roll Accel/1, Discrete-Time Integrator1/1
  Discrete-Time Integrator1/1 -> Discrete-Time Integrator/1, roll_rate/1, [RollRate]

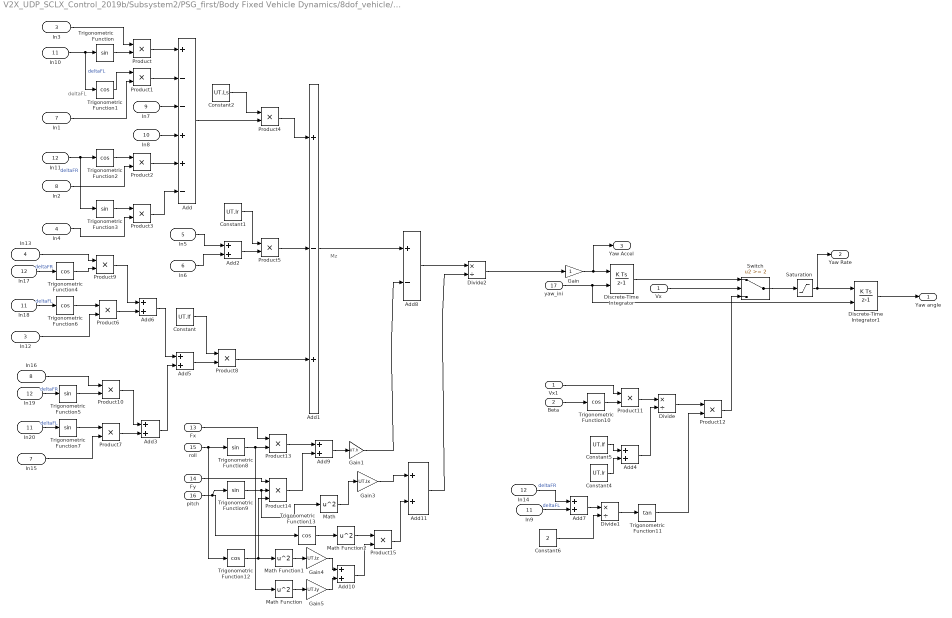
== system V2X_UDP_SCLX_Control_2019b/Subsystem2/PSG_first/Body Fixed Vehicle Dynamics/8dof_vehicle/Yaw Dynamics ==
  note: Mz
  note: deltaFL
  Vx : Inport
  Beta : Inport  Port=2
  In3 : Inport  Port=3
  In4 : Inport  Port=4
  In5 : Inport  Port=5
  In6 : Inport  Port=6
  In1 : Inport  Port=7
  In2 : Inport  Port=8
  In7 : Inport  Port=9
  In8 : Inport  Port=10
  In10 : Inport  Port=11
  In11 : Inport  Port=12
  Fx : Inport  Port=13
  Fy : Inport  Port=14
  roll : Inport  Port=15
  "pitch " : Inport  Port=16
  yaw_ini : Inport  Port=17
  Add : Sum  Inputs=+--++-
  Add1 : Sum  Inputs=+-+
  Add{2..7,9..11} (9 alike) : Sum
  Add8 : Sum  Inputs=+-
  Constant : Constant  Value=UT.lf
  Constant1 : Constant  Value=UT.lr
  Constant2 : Constant  Value=UT.Ls
  Constant4 : Constant  Value=UT.lr
  Constant5 : Constant  Value=UT.lf
  Constant6 : Constant  Value=2
  Discrete-Time Integrator : DiscreteIntegrator  InitialConditionSource=external  InitialCondition=UT.Veh_PSG_o(3)  SampleTime=UT.Ts_Veh  ICPrevOutput=DiscIntNeverNeededParam  ICPrevScaledInput=DiscIntNeverNeededParam
  Discrete-Time Integrator1 : DiscreteIntegrator  InitialConditionSource=external  InitialCondition=UT.Veh_PSG_o(3)  SampleTime=UT.Ts_Veh  ICPrevOutput=DiscIntNeverNeededParam  ICPrevScaledInput=DiscIntNeverNeededParam
  Divide : Product  Inputs=*/
  Divide1 : Product  Inputs=*/
  Divide2 : Product  Inputs=*/
  Gain : Gain
  Gain1 : Gain  Gain=UT.h
  Gain3 : Gain  Gain=UT.Ix
  Gain4 : Gain  Gain=UT.Iz
  Gain5 : Gain  Gain=UT.Iy
  In12 : InportShadow  Port=3
  In13 : InportShadow  Port=4
  In14 : InportShadow  Port=12
  In15 : InportShadow  Port=7
  In16 : InportShadow  Port=8
  In17 : InportShadow  Port=12
  In18 : InportShadow  Port=11
  In19 : InportShadow  Port=12
  In20 : InportShadow  Port=11
  In9 : InportShadow  Port=11
  "Math " : Math  Operator=square  SignedPower=on  SaturateOnIntegerOverflow=on
  Math Function : Math  Operator=square  SignedPower=on  SaturateOnIntegerOverflow=on
  Math Function1 : Math  Operator=square  SignedPower=on  SaturateOnIntegerOverflow=on
  Math Function2 : Math  Operator=square  SignedPower=on  SaturateOnIntegerOverflow=on
  Product{,1..13,15} (15 alike) : Product
  Product14 : Product  Inputs=3
  Saturation : Saturate  UpperLimit=50*3.14/180  LowerLimit=-50*3.14/180  SampleTime=UT.Ts_Veh
  Switch : Switch  Threshold=2
  Trigonometric Function{,3,5,7..9} (6 alike) : Trigonometry
  Trigonometric Function{1..2,4,6,10,12..13} (7 alike) : Trigonometry  Operator=cos
  Trigonometric Function11 : Trigonometry  Operator=tan
  Vx1 : InportShadow
  Yaw angle : Outport  VectorParamsAs1DForOutWhenUnconnected=off
  Yaw Rate : Outport  Port=2  VectorParamsAs1DForOutWhenUnconnected=off
  Yaw Accel : Outport  Port=3  VectorParamsAs1DForOutWhenUnconnected=off
  wires:
  yaw_ini/1 -> Discrete-Time Integrator1/2, Discrete-Time Integrator/2
  Discrete-Time Integrator/1 -> Switch/1
  Discrete-Time Integrator1/1 -> Yaw angle/1
  Gain/1 -> Yaw Accel/1, Discrete-Time Integrator/1
  Vx/1 -> Switch/2
  Constant4/1 -> Add4/2
  Constant5/1 -> Add4/1
  Add4/1 -> Divide/2
  Add7/1 -> Divide1/1
  Constant6/1 -> Divide1/2
  Beta/1 -> Trigonometric Function10/1
  Vx1/1 -> Product11/1
  Trigonometric Function10/1 -> Product11/2
  Product11/1 -> Divide/1
  Divide1/1 -> Trigonometric Function11/1
  Trigonometric Function11/1 -> Product12/2
  Divide/1 -> Product12/1
  Switch/1 -> Saturation/1
  Product12/1 -> Switch/3
  Saturation/1 -> Discrete-Time Integrator1/1, Yaw Rate/1
  In10/1 -> Trigonometric Function1/1, Trigonometric Function/1  "deltaFL"
  In3/1 -> Product/1
  Trigonometric Function/1 -> Product/2
  Product/1 -> Add/1
  Trigonometric Function1/1 -> Product1/1
  In1/1 -> Product1/2
  Product1/1 -> Add/2
  In7/1 -> Add/3
  In8/1 -> Add/4
  Trigonometric Function2/1 -> Product2/1
  In2/1 -> Product2/2
  Product2/1 -> Add/5
  Trigonometric Function3/1 -> Product3/1
  In4/1 -> Product3/2
  Product3/1 -> Add/6
  Add/1 -> Product4/2
  Constant2/1 -> Product4/1
  Product4/1 -> Add1/1
  In5/1 -> Add2/1
  In6/1 -> Add2/2
  Add2/1 -> Product5/2
  Constant1/1 -> Product5/1
  Product5/1 -> Add1/2
  In13/1 -> Product9/1
  Add1/1 -> Add8/1
  Add6/1 -> Add5/1
  Add5/1 -> Product8/2
  Constant/1 -> Product8/1
  Product8/1 -> Add1/3
  In11/1 -> Trigonometric Function3/1, Trigonometric Function2/1  "deltaFR"
  In12/1 -> Product6/2
  Product9/1 -> Add6/1
  Product6/1 -> Add6/2
  Trigonometric Function4/1 -> Product9/2
  Trigonometric Function6/1 -> Product6/1
  In18/1 -> Trigonometric Function6/1  "deltaFL"
  In17/1 -> Trigonometric Function4/1  "deltaFR"
  In16/1 -> Product10/1
  Add3/1 -> Add5/2
  In15/1 -> Product7/2
  Product10/1 -> Add3/1
  Product7/1 -> Add3/2
  Trigonometric Function5/1 -> Product10/2
  Trigonometric Function7/1 -> Product7/1
  In19/1 -> Trigonometric Function5/1  "deltaFR"
  In20/1 -> Trigonometric Function7/1  "deltaFL"
  In9/1 -> Add7/2  "deltaFL"
  In14/1 -> Add7/1  "deltaFR"
  roll/1 -> Trigonometric Function8/1, Trigonometric Function12/1
  Trigonometric Function8/1 -> Math Function/1, Product13/2
  Fx/1 -> Product13/1
  Product13/1 -> Add9/1
  Fy/1 -> Product14/1
  "pitch "/1 -> Trigonometric Function9/1, Trigonometric Function13/1
  Trigonometric Function9/1 -> "Math "/1, Product14/2
  Trigonometric Function12/1 -> Product14/3, Math Function1/1
  Product14/1 -> Add9/2
  Add9/1 -> Gain1/1
  Gain1/1 -> Add8/2
  Add8/1 -> Divide2/1
  Math Function/1 -> Gain5/1
  Gain5/1 -> Add10/2
  Math Function1/1 -> Gain4/1
  Gain4/1 -> Add10/1
  Add10/1 -> Product15/2
  Trigonometric Function13/1 -> Math Function2/1
  Math Function2/1 -> Product15/1
  Product15/1 -> Add11/2
  Gain3/1 -> Add11/1
  "Math "/1 -> Gain3/1
  Add11/1 -> Divide2/2
  Divide2/1 -> Gain/1

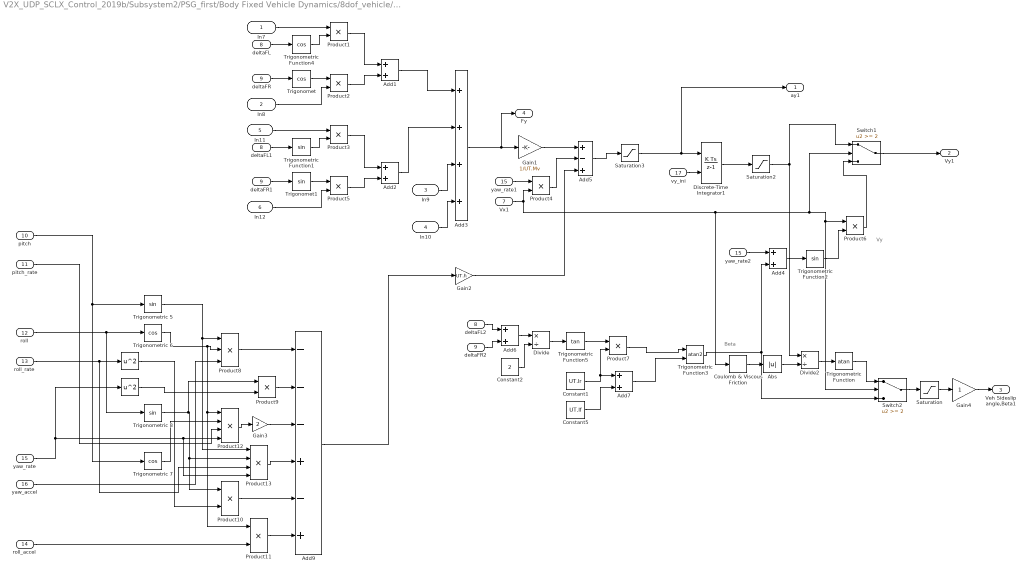
== system V2X_UDP_SCLX_Control_2019b/Subsystem2/PSG_first/Body Fixed Vehicle Dynamics/8dof_vehicle/lateral ==
  note: Beta
  note: Vy
  In7 : Inport
  In8 : Inport  Port=2
  In9 : Inport  Port=3
  In10 : Inport  Port=4
  In11 : Inport  Port=5
  In12 : Inport  Port=6
  Vx1 : Inport  Port=7
  deltaFL : Inport  Port=8
  deltaFR : Inport  Port=9
  pitch : Inport  Port=10
  pitch_rate : Inport  Port=11
  roll : Inport  Port=12
  roll_rate : Inport  Port=13
  roll_accel : Inport  Port=14
  yaw_rate : Inport  Port=15
  yaw_accel : Inport  Port=16
  vy_ini : Inport  Port=17
  " " : Math  Operator=square  SignedPower=on  SaturateOnIntegerOverflow=on
  " " : Math  Operator=square  SignedPower=on  SaturateOnIntegerOverflow=on
  Abs : Abs
  Add{1..2,4,6..7} (5 alike) : Sum
  Add3 : Sum  Inputs=++++
  Add5 : Sum  Inputs=+-+
  Add9 : Sum  Inputs=---+-+
  Constant1 : Constant  Value=UT.lr
  Constant2 : Constant  Value=2
  Constant5 : Constant  Value=UT.lf
  Coulomb & Viscous Friction : simulink/Discontinuities/Coulomb & Viscous Friction  offset=0.01  gain=1
  Discrete-Time Integrator1 : DiscreteIntegrator  InitialConditionSource=external  InitialCondition=UT.Veh_PSG_o(2)  SampleTime=UT.Ts_Veh  ICPrevOutput=DiscIntNeverNeededParam  ICPrevScaledInput=DiscIntNeverNeededParam
  Divide : Product  Inputs=*/
  Divide2 : Product  Inputs=*/
  Gain1 : Gain  Gain=1/UT.Mv
  Gain2 : Gain  Gain=UT.h
  Gain3 : Gain  Gain=2
  Gain4 : Gain
  Product{1..3,5..7,9..11} (9 alike) : Product
  Product12 : Product  Inputs=4
  Product13 : Product  Inputs=4
  Product4 : Product  RndMeth=Zero
  Product8 : Product  Inputs=3
  Saturation : Saturate  UpperLimit=10*3.14/180  LowerLimit=-10*3.14/180
  Saturation2 : Saturate  UpperLimit=100  LowerLimit=-100
  Saturation3 : Saturate  UpperLimit=6  LowerLimit=-6
  Switch1 : Switch  Threshold=2
  Switch2 : Switch  Threshold=2
  Trigonomet : Trigonometry  Operator=cos
  Trigonomet1 : Trigonometry
  Trigonometric 5 : Trigonometry
  Trigonometric 6 : Trigonometry  Operator=cos
  Trigonometric 7 : Trigonometry  Operator=cos
  Trigonometric 8 : Trigonometry
  Trigonometric Function : Trigonometry  Operator=atan
  Trigonometric Function1 : Trigonometry
  Trigonometric Function2 : Trigonometry
  Trigonometric Function3 : Trigonometry  Operator=atan2
  Trigonometric Function4 : Trigonometry  Operator=cos
  Trigonometric Function5 : Trigonometry  Operator=tan
  deltaFL1 : InportShadow  Port=8
  deltaFL2 : InportShadow  Port=8
  deltaFR1 : InportShadow  Port=9
  deltaFR2 : InportShadow  Port=9
  yaw_rate1 : InportShadow  Port=15
  yaw_rate2 : InportShadow  Port=15
  ay1 : Outport  VectorParamsAs1DForOutWhenUnconnected=off
  Vy1 : Outport  Port=2  VectorParamsAs1DForOutWhenUnconnected=off
  Veh Sideslip angle,Beta1 : Outport  Port=3  VectorParamsAs1DForOutWhenUnconnected=off
  Fy : Outport  Port=4  VectorParamsAs1DForOutWhenUnconnected=off
  wires:
  vy_ini/1 -> Discrete-Time Integrator1/2
  Gain1/1 -> Add5/1
  Add5/1 -> Saturation3/1
  In7/1 -> Product1/1
  In8/1 -> Product2/2
  yaw_rate1/1 -> Product4/1
  Add1/1 -> Add3/1
  In9/1 -> Add3/3
  In10/1 -> Add3/4
  Product4/1 -> Add5/2
  Discrete-Time Integrator1/1 -> Saturation2/1
  Trigonomet/1 -> Product2/1
  Trigonometric Function4/1 -> Product1/2
  deltaFL/1 -> Trigonometric Function4/1
  deltaFR/1 -> Trigonomet/1
  Product1/1 -> Add1/1
  Product2/1 -> Add1/2
  In11/1 -> Product3/1
  In12/1 -> Product5/2
  Trigonomet1/1 -> Product5/1
  Trigonometric Function1/1 -> Product3/2
  Product3/1 -> Add2/1
  Product5/1 -> Add2/2
  Add2/1 -> Add3/2
  deltaFL1/1 -> Trigonometric Function1/1
  deltaFR1/1 -> Trigonomet1/1
  yaw_rate2/1 -> Add4/1
  Add4/1 -> Trigonometric Function2/1
  Trigonometric Function2/1 -> Product6/2
  deltaFL2/1 -> Add6/1
  deltaFR2/1 -> Add6/2
  Add6/1 -> Divide/1
  Constant2/1 -> Divide/2
  Divide/1 -> Trigonometric Function5/1
  Trigonometric Function5/1 -> Product7/1
  Constant1/1 -> Product7/2, Add7/1
  Product7/1 -> Trigonometric Function3/1
  Constant5/1 -> Add7/2
  Saturation2/1 -> Divide2/1, Switch1/1
  Product6/1 -> Switch1/3
  Divide2/1 -> Trigonometric Function/1
  Trigonometric Function3/1 -> Add4/2, Switch2/3
  Vx1/1 -> Product4/2, Coulomb & Viscous Friction/1, Product6/1, Switch2/2, Switch1/2
  Abs/1 -> Divide2/2
  Add7/1 -> Trigonometric Function3/2
  Switch2/1 -> Saturation/1
  Saturation/1 -> Gain4/1
  Gain2/1 -> Add5/3
  pitch_rate/1 -> Product12/3
  roll_rate/1 -> Product13/3, " "/1
  yaw_rate/1 -> Product13/4, Product12/4, " "/1
  yaw_accel/1 -> Product8/3
  pitch/1 -> Trigonometric 7/1, Trigonometric 5/1
  roll/1 -> Trigonometric 8/1, Trigonometric 6/1
  Trigonometric 6/1 -> Product11/1, Product12/1, Product8/2
  Trigonometric 5/1 -> Product13/1, Product8/1
  Product8/1 -> Add9/1
  Product9/1 -> Add9/2
  Product12/1 -> Gain3/1
  Gain3/1 -> Add9/3
  Trigonometric 7/1 -> Product12/2
  Product13/1 -> Add9/4
  Product10/1 -> Add9/5
  Trigonometric 8/1 -> Product9/1, Product13/2, Product10/1
  Product11/1 -> Add9/6
  " "/1 -> Product9/2
  " "/1 -> Product10/2
  roll_accel/1 -> Product11/2
  Trigonometric Function/1 -> Switch2/1
  Add3/1 -> Fy/1, Gain1/1
  Add9/1 -> Gain2/1
  Gain4/1 -> Veh Sideslip angle,Beta1/1
  Saturation3/1 -> Discrete-Time Integrator1/1, ay1/1
  Switch1/1 -> Vy1/1
  Coulomb & Viscous Friction/1 -> Abs/1

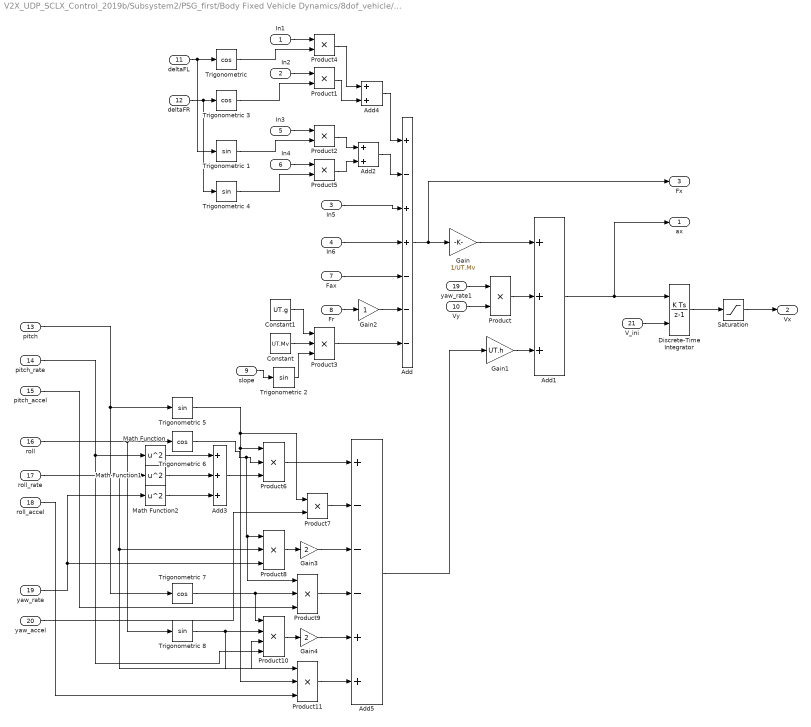
== system V2X_UDP_SCLX_Control_2019b/Subsystem2/PSG_first/Body Fixed Vehicle Dynamics/8dof_vehicle/longitudinal ==
  In1 : Inport
  In2 : Inport  Port=2
  In5 : Inport  Port=3
  In6 : Inport  Port=4
  In3 : Inport  Port=5
  In4 : Inport  Port=6
  Fax : Inport  Port=7
  Fr : Inport  Port=8
  slope : Inport  Port=9
  Vy : Inport  Port=10
  deltaFL : Inport  Port=11
  deltaFR : Inport  Port=12
  pitch : Inport  Port=13
  pitch_rate : Inport  Port=14
  pitch_accel : Inport  Port=15
  roll : Inport  Port=16
  roll_rate : Inport  Port=17
  roll_accel : Inport  Port=18
  yaw_rate : Inport  Port=19
  yaw_accel : Inport  Port=20
  V_ini : Inport  Port=21
  Add : Sum  Inputs=+-++---
  Add1 : Sum  Inputs=+++
  Add2 : Sum
  Add3 : Sum  Inputs=+++
  Add4 : Sum
  Add5 : Sum  Inputs=+---++
  Constant : Constant  Value=UT.Mv
  Constant1 : Constant  Value=UT.g
  Discrete-Time Integrator : DiscreteIntegrator  InitialConditionSource=external  InitialCondition=UT.Veh_PSG_o(1)  SampleTime=UT.Ts_Veh  ICPrevOutput=DiscIntNeverNeededParam  ICPrevScaledInput=DiscIntNeverNeededParam
  Gain : Gain  Gain=1/UT.Mv
  Gain1 : Gain  Gain=UT.h
  Gain2 : Gain
  Gain3 : Gain  Gain=2
  Gain4 : Gain  Gain=2
  Math Function : Math  Operator=square  SignedPower=on  SaturateOnIntegerOverflow=on
  Math Function1 : Math  Operator=square  SignedPower=on  SaturateOnIntegerOverflow=on
  Math Function2 : Math  Operator=square  SignedPower=on  SaturateOnIntegerOverflow=on
  Product{,1..2,4..5,7} (6 alike) : Product
  Product10 : Product  Inputs=4
  Product{3,6,8..9,11} (5 alike) : Product  Inputs=3
  Saturation : Saturate  UpperLimit=50  LowerLimit=0
  Trigonometric {,3,6..7} (4 alike) : Trigonometry  Operator=cos
  Trigonometric {1..2,4..5,8} (5 alike) : Trigonometry
  yaw_rate1 : InportShadow  Port=19
  ax : Outport  VectorParamsAs1DForOutWhenUnconnected=off
  Vx : Outport  Port=2  VectorParamsAs1DForOutWhenUnconnected=off
  Fx : Outport  Port=3  VectorParamsAs1DForOutWhenUnconnected=off
  wires:
  V_ini/1 -> Discrete-Time Integrator/2
  Discrete-Time Integrator/1 -> Saturation/1
  Fax/1 -> Add/5
  Fr/1 -> Gain2/1
  slope/1 -> Trigonometric 2/1
  Product3/1 -> Add/7
  yaw_rate1/1 -> Product/1
  Vy/1 -> Product/2
  Add/1 -> Fx/1, Gain/1
  Product/1 -> Add1/2
  Gain/1 -> Add1/1
  In1/1 -> Product4/1
  Product4/1 -> Add4/1
  Add4/1 -> Add/1
  In3/1 -> Product2/1
  In4/1 -> Product5/1
  Add2/1 -> Add/2
  In5/1 -> Add/3
  In6/1 -> Add/4
  Add1/1 -> Discrete-Time Integrator/1, ax/1
  Trigonometric 2/1 -> Product3/3
  Constant1/1 -> Product3/1
  Constant/1 -> Product3/2
  Gain2/1 -> Add/6
  Product1/1 -> Add4/2
  In2/1 -> Product1/1
  deltaFL/1 -> Trigonometric 1/1, "Trigonometric "/1
  "Trigonometric "/1 -> Product4/2
  deltaFR/1 -> Trigonometric 4/1, Trigonometric 3/1
  Trigonometric 3/1 -> Product1/2
  Trigonometric 1/1 -> Product2/2
  Trigonometric 4/1 -> Product5/2
  Product2/1 -> Add2/1
  Product5/1 -> Add2/2
  Saturation/1 -> Vx/1
  Gain1/1 -> Add1/3
  pitch_rate/1 -> Product10/4, Math Function/1
  roll_rate/1 -> Product10/3, Product8/2, Math Function1/1
  yaw_rate/1 -> Product8/3, Math Function2/1
  Math Function/1 -> Add3/1
  Math Function1/1 -> Add3/2
  Math Function2/1 -> Add3/3
  Add3/1 -> Product6/3
  pitch/1 -> Trigonometric 7/1, Trigonometric 5/1
  roll/1 -> Trigonometric 8/1, Trigonometric 6/1
  Trigonometric 6/1 -> Product9/1, Product8/1, Product6/2
  Trigonometric 5/1 -> Product7/1, Product11/2, Product6/1
  Product6/1 -> Add5/1
  yaw_accel/1 -> Product7/2
  Product7/1 -> Add5/2
  Product8/1 -> Gain3/1
  Gain3/1 -> Add5/3
  Trigonometric 7/1 -> Product10/1, Product9/2
  pitch_accel/1 -> Product9/3
  Product9/1 -> Add5/4
  Gain4/1 -> Add5/5
  Product10/1 -> Gain4/1
  Trigonometric 8/1 -> Product11/1, Product10/2
  Product11/1 -> Add5/6
  roll_accel/1 -> Product11/3
  Add5/1 -> Gain1/1

== system V2X_UDP_SCLX_Control_2019b/Subsystem2/PSG_first/Body Fixed Vehicle Dynamics/Driving Resistance Subsystem/Aerodynamic Resistance ==
  note: Fa=0.5*p*Cd*A(Vx+Vw)^2
  note: Vx=m/s
  note: increaesd to 0.75*...
  Vx : Inport
  X Aerodynamic Fcn : Fcn  Expr=0.75*UT.rho*UT.Cd*UT.Awind*(u(1)+UT.Vw)^2  SampleTime=UT.Ts_Veh
  Fa : Outport  VectorParamsAs1DForOutWhenUnconnected=off
  wires:
  X Aerodynamic Fcn/1 -> Fa/1
  Vx/1 -> X Aerodynamic Fcn/1

== system V2X_UDP_SCLX_Control_2019b/Subsystem2/PSG_first/Body Fixed Vehicle Dynamics/Driving Resistance Subsystem/Rolling resistance ==
  note: added *2
  Vx : Inport
  Rolling resistance Fcn1 : Fcn  Expr=(0.005+(1/2.013)*(0.01+0.0095*((3.6*u(1))/100)^2))*UT.Mv*UT.g*2  SampleTime=UT.Ts_Veh
  Fr : Outport  VectorParamsAs1DForOutWhenUnconnected=off
  wires:
  Vx/1 -> Rolling resistance Fcn1/1
  Rolling resistance Fcn1/1 -> Fr/1

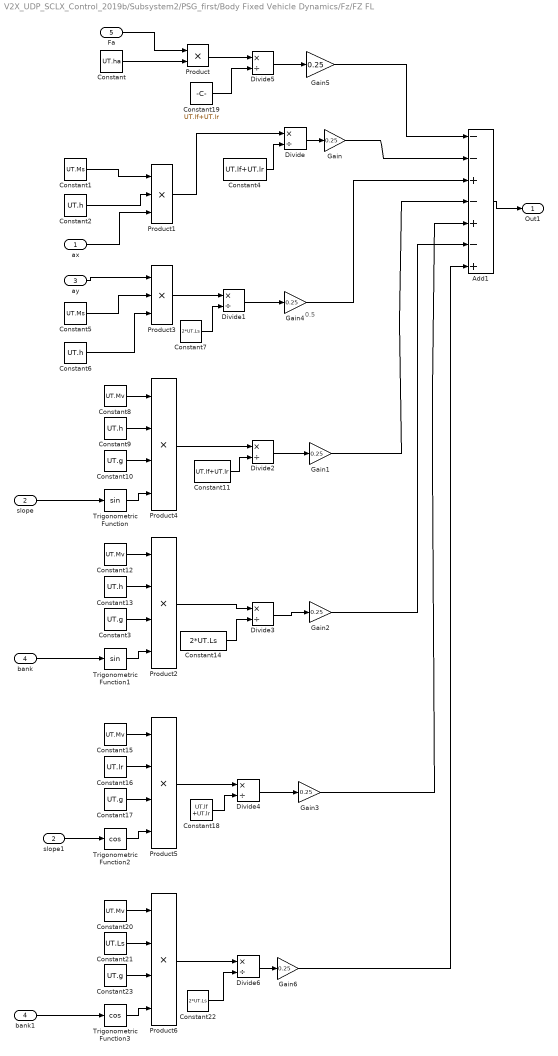
== system V2X_UDP_SCLX_Control_2019b/Subsystem2/PSG_first/Body Fixed Vehicle Dynamics/Fz/FZ FL ==
  note: 0.5
  ax : Inport
  slope : Inport  Port=2
  ay : Inport  Port=3
  bank : Inport  Port=4
  Fa : Inport  Port=5
  Add1 : Sum  Inputs=--+-+-+
  Constant : Constant  Value=UT.ha
  Constant1 : Constant  Value=UT.Ms
  Constant{3,10,17,23} (4 alike) : Constant  Value=UT.g
  Constant11 : Constant  Value=UT.lf+UT.lr
  Constant{8,12,15,20} (4 alike) : Constant  Value=UT.Mv
  Constant{2,6,9,13} (4 alike) : Constant  Value=UT.h
  Constant14 : Constant  Value=2*UT.Ls
  Constant16 : Constant  Value=UT.lr
  Constant18 : Constant  Value=UT.lf +UT.lr
  Constant19 : Constant  Value=UT.lf+UT.lr
  Constant21 : Constant  Value=UT.Ls
  Constant22 : Constant  Value=2*UT.Ls
  Constant4 : Constant  Value=UT.lf+UT.lr
  Constant5 : Constant  Value=UT.Ms
  Constant7 : Constant  Value=2*UT.Ls
  Divide{,1..6} (7 alike) : Product  Inputs=*/
  Gain{,1..6} (7 alike) : Gain  Gain=0.25
  Product : Product
  Product1 : Product  Inputs=3
  Product{2,4..6} (4 alike) : Product  Inputs=4
  Product3 : Product  Inputs=3
  Trigonometric Function : Trigonometry
  Trigonometric Function1 : Trigonometry
  Trigonometric Function2 : Trigonometry  Operator=cos
  Trigonometric Function3 : Trigonometry  Operator=cos
  bank1 : InportShadow  Port=4
  slope1 : InportShadow  Port=2
  Out1 : Outport  VectorParamsAs1DForOutWhenUnconnected=off
  wires:
  Constant1/1 -> Product1/1
  Constant2/1 -> Product1/2
  ax/1 -> Product1/3
  Constant4/1 -> Divide/2
  ay/1 -> Product3/1
  Constant5/1 -> Product3/2
  Constant6/1 -> Product3/3
  Product3/1 -> Divide1/1
  Constant7/1 -> Divide1/2
  Divide/1 -> Gain/1
  Divide1/1 -> Gain4/1
  Constant8/1 -> Product4/1
  Constant9/1 -> Product4/2
  Constant10/1 -> Product4/3
  slope/1 -> Trigonometric Function/1
  Trigonometric Function/1 -> Product4/4
  Constant11/1 -> Divide2/2
  Divide2/1 -> Gain1/1
  Product4/1 -> Divide2/1
  Constant12/1 -> Product2/1
  Constant13/1 -> Product2/2
  Constant3/1 -> Product2/3
  bank/1 -> Trigonometric Function1/1
  Trigonometric Function1/1 -> Product2/4
  Product2/1 -> Divide3/1
  Constant14/1 -> Divide3/2
  Divide3/1 -> Gain2/1
  Constant15/1 -> Product5/1
  Constant16/1 -> Product5/2
  Constant17/1 -> Product5/3
  Trigonometric Function2/1 -> Product5/4
  slope1/1 -> Trigonometric Function2/1
  Constant18/1 -> Divide4/2
  Product5/1 -> Divide4/1
  Divide4/1 -> Gain3/1
  Add1/1 -> Out1/1
  Product1/1 -> Divide/1
  Fa/1 -> Product/1
  Constant/1 -> Product/2
  Product/1 -> Divide5/1
  Constant19/1 -> Divide5/2
  Divide5/1 -> Gain5/1
  Gain5/1 -> Add1/1
  Gain/1 -> Add1/2
  Gain1/1 -> Add1/4
  Gain3/1 -> Add1/5
  Gain4/1 -> Add1/3
  Gain2/1 -> Add1/6
  Constant20/1 -> Product6/1
  Constant21/1 -> Product6/2
  Constant23/1 -> Product6/3
  bank1/1 -> Trigonometric Function3/1
  Trigonometric Function3/1 -> Product6/4
  Product6/1 -> Divide6/1
  Constant22/1 -> Divide6/2
  Divide6/1 -> Gain6/1
  Gain6/1 -> Add1/7
